simulink model "kinematic_bicycle_model"  (R2022b)
settings: Solver=VariableStepAuto  StartTime=0.0  StopTime=3  RelTol=1e-3
undefined symbols (not defined in the file): lf, lr, Vx
libraries: simulink_extras x1
settings Model: Creator=Timothy  LastModifiedBy=Timothy

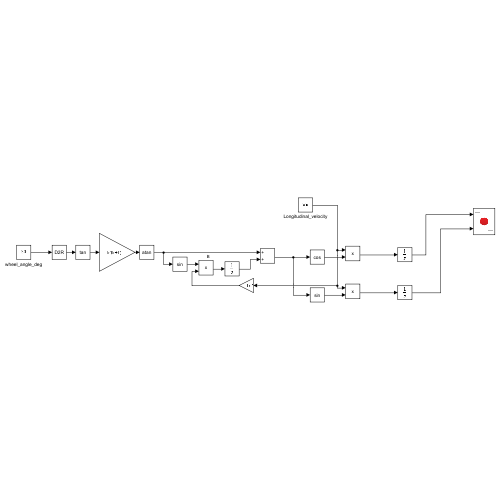
[thumbnail: Simulink's stored preview of the top-level diagram]
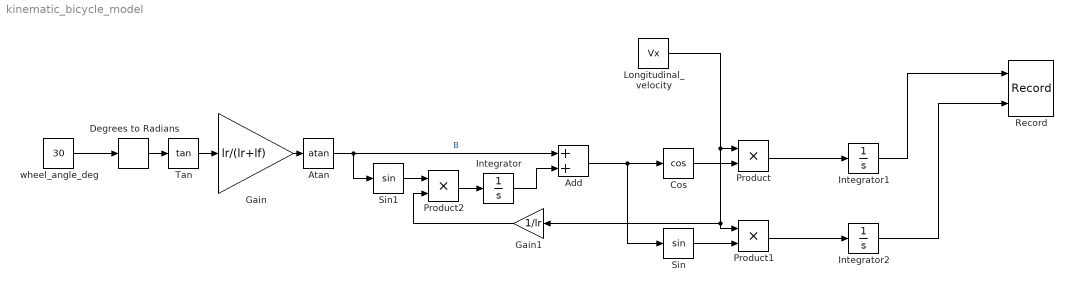
== system kinematic_bicycle_model ==
  Add : Sum
  Atan : Trigonometry  Operator=atan
  Cos : Trigonometry  Operator=cos
  Degrees to Radians : simulink_extras/Transformations/Degrees to Radians
  Gain : Gain  Gain=lr/(lr+lf)
  Gain1 : Gain  Gain=1/lr
  Integrator : Integrator
  Integrator1 : Integrator
  Integrator2 : Integrator
  Longitudinal_velocity : Constant  Value=Vx
  Product : Product
  Product1 : Product
  Product2 : Product
  Record : Record  FileSettingsInternal="{\"entries\":[{\"content\":{\"excelSettings\":{\"content\":{},\"type\":\"Streamout.ExcelSettings\"}},\"type\":\"Streamout.FileSettingStorage\",\"uuid\":\"1fc89837-2e6e-4cfe-af64-4bb95cf763e5\"}],\"packageUris\":[\"http://schema.mathworks.com/mf0/streamout_blocks/R2020a\"],\"version\":\"1.0\"}"  Layout=[1 1]  SignalsInternal="{\"entries\":[{\"content\":{\"signals\":[{\"content\":{\"blockPath\":[\"kinematic_bicycle_model/Record\"],\"channel\":[],\"dimensions\":[1],\"domain\":\"kinematic_bicycle_model/Record\",\"lineColor\":\"#4dbeee\",\"plots\":[1],\"port\":1,\"sid\":[\"\"],\"signalID\":2941,\"signalName\":\"Integrator1\"},\"type\":\"RecordBlkView.Signal\",\"uuid\":\"75d96448-8392-4039-ae92-9a209dd0feac\"},{\"content\":{\"blockPath\":[\"kinematic_bicycle_model/Record\"],\"channel\":[],\"dimensions\":[1],\"domain\":\"kinematic_bicycle_model/Record\",\"lineColor\":\"#a2142f\",\"plots\":[1],\"port\":2,\"sid\":[\"\"],\"signalID\":2945,\"signalName\":\"Integrator2\"},\"type\":\"RecordBlkView.Signal\",\"uuid\":\"3a0f78d1-ba60-4f29-8a3e-3bccc9555ea3\"}]},\"type\":\"RecordBlkView.InputSignals\",\"uuid\":\"a341f0b6-2848-4ad9-9028-cd6a8ac371e6\"}],\"packageUris\":[\"http://schema.mathworks.com/mf0/streamout_blocks/R2020a\"],\"version\":\"1.0\"}"  VisualizationBindings="{\"xyplotplugin\":{\"info\":[{\"series\":[{\"bindingParametersList\":[{\"parameter\":\"Y-Axis\",\"signalID\":2945,\"signalName\":\"Integrator2\"},{\"parameter\":\"X-Axis\",\"signalID\":2941,\"signalName\":\"Integrator1\"}],\"seriesID\":643}],\"subplotID\":1}]}}"
  Sin : Trigonometry
  Sin1 : Trigonometry
  Tan : Trigonometry  Operator=tan
  wheel_angle_deg : Constant  Value=30
  wires:
  Add/1 -> Sin/1, Cos/1
  Atan/1 -> Add/1, Sin1/1  "B"
  Tan/1 -> Gain/1
  wheel_angle_deg/1 -> Degrees to Radians/1
  Gain/1 -> Atan/1
  Degrees to Radians/1 -> Tan/1
  Cos/1 -> Product/2
  Product/1 -> Integrator1/1
  Longitudinal_velocity/1 -> Product1/1, Gain1/1, Product/1
  Sin/1 -> Product1/2
  Product1/1 -> Integrator2/1
  Sin1/1 -> Product2/1
  Gain1/1 -> Product2/2
  Product2/1 -> Integrator/1
  Integrator/1 -> Add/2
  Integrator1/1 -> Record/1
  Integrator2/1 -> Record/2
